simulink model "model_test"  (R2023b)
settings: Solver=FixedStepAuto  StartTime=0.0  StopTime=10.0  RelTol=1e-3
settings Model: Creator=Tsmc  LastModifiedBy=Tsmc
settings OptimizationCC: DefaultParameterBehavior=Inlined

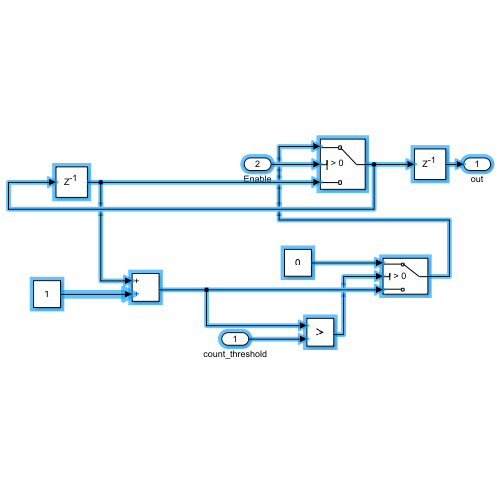
[thumbnail: Simulink's stored preview of the top-level diagram]
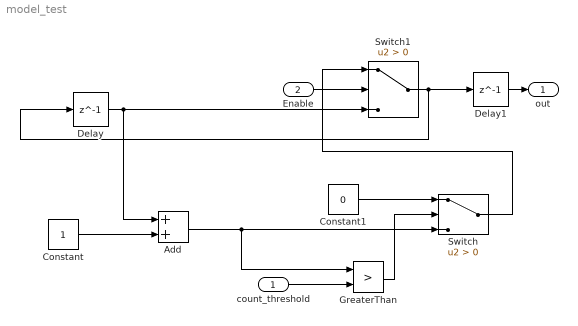
== system model_test ==
  count_threshold : Inport
  Enable : Inport  Port=2
  Add : Sum  AccumDataTypeStr=uint8
  Constant : Constant  OutDataTypeStr=uint8
  Constant1 : Constant  Value=0  OutDataTypeStr=uint8
  Delay : Delay  DelayLength=1
  Delay1 : Delay  DelayLength=1
  GreaterThan : RelationalOperator  Operator=>  OutDataTypeStr=boolean  RndMeth=Simplest  InputSameDT=off
  Switch : Switch  Criteria=u2 > Threshold  SaturateOnIntegerOverflow=off  InputSameDT=off
  Switch1 : Switch  Criteria=u2 > Threshold  SaturateOnIntegerOverflow=off  InputSameDT=off
  out : Outport  VectorParamsAs1DForOutWhenUnconnected=off
  wires:
  Enable/1 -> Switch1/2
  Switch1/1 -> Delay1/1, Delay/1
  Switch/1 -> Switch1/1
  Delay1/1 -> out/1
  GreaterThan/1 -> Switch/2
  Delay/1 -> Add/1, Switch1/3
  Add/1 -> GreaterThan/1, Switch/3
  count_threshold/1 -> GreaterThan/2
  Constant1/1 -> Switch/1
  Constant/1 -> Add/2
